simulink model "SimulinkAnalysisofCheetahTail"  (R2022a)
settings: Solver=ode4  StartTime=0.0  StopTime=1.5  FixedStep=0.001  RelTol=1e-3
undefined symbols (not defined in the file): B_cg_H, B_con_H, B_con_L, bar_len, cd_table, Cf, cl_table, g, gear_ratio, int_point_bar, int_point_tail, ITail, M_add, M_cg_H, M_cg_L, M_cg_W, Mb, Mm, Mt, psi3, rho, T_cg_H, T_fur_gap, T_length, T_width_major, T_width_minor, th2_initial, torque_constant, uncertainty_Forces, uncertainty_Position, Vf, windspeed
(part 10 of 21)

== matlab function SimulinkAnalysisofCheetahTail/Model/MassMatrix ==
  data: B_cg_H parameter; B_con_H parameter; B_con_L parameter; ITail parameter; M_cg_H parameter; M_cg_L parameter; M_cg_W parameter; Mb parameter; Mm parameter; Mt parameter; T_cg_H parameter; MassMatrix output; q input
function MassMatrix = MassMatrix(B_cg_H,B_con_H,B_con_L,ITail,M_cg_H,M_cg_L,M_cg_W,Mb,Mm,Mt,T_cg_H,q)
%#codegen
[x,y,z,phi1,th1,psi1,phi2,th2] = deal(q(1),q(2),q(3),q(4),q(5),q(6),q(7),q(8));
% [dx,dy,dz,dphi1,dth1,dpsi1,dphi2,dth2] = deal(dq(1),dq(2),dq(3),dq(4),dq(5),dq(6),dq(7),dq(8));
%    This function was generated by the Symbolic Math Toolbox version 9.0.
%    26-Jan-2022 10:16:26

t2 = cos(phi1);
t3 = cos(phi2);
t4 = cos(psi1);
t5 = cos(th1);
t6 = cos(th2);
t7 = sin(phi1);
t8 = sin(phi2);
t9 = sin(psi1);
t10 = sin(th1);
t11 = sin(th2);
t12 = M_cg_L+x;
t13 = M_cg_W+y;
t14 = M_cg_H+z;
t15 = B_cg_H.^2;
t16 = t2.^2;
t17 = t4.^2;
t18 = t5.^2;
t19 = t7.^2;
t20 = t9.^2;
t21 = t10.^2;
t22 = B_con_L.*t5;
t23 = t2.*t4;
t24 = t5.*t6;
t25 = t2.*t8;
t26 = t2.*t9;
t27 = t4.*t7;
t28 = t6.*t10;
t29 = t7.*t9;
t30 = t10.*t11;
t32 = t5.*t12;
t33 = B_con_H.*t2.*t10;
t34 = B_con_H.*t5.*t7;
t35 = B_con_L.*t4.*t10;
t37 = B_con_L.*t9.*t10;
t40 = t5.*t8.*t11;
t42 = t5.*t9.*t11;
t44 = t7.*t8.*t10;
t48 = t2.*t3.*t5;
t52 = t3.*t5.*t7;
t53 = t3.*t6.*t7;
t55 = t2.*t5.*t11;
t56 = t3.*t5.*t11;
t58 = t4.*t5.*t11;
t61 = t3.*t7.*t10;
t62 = t5.*t7.*t8;
t68 = t2.*t5.*t13;
t70 = t4.*t10.*t12;
t72 = Mb.*t2.*t5.*t10;
t73 = Mm.*t2.*t5.*t10;
t74 = Mt.*t2.*t5.*t10;
t75 = t2.*t10.*t14;
t76 = t5.*t7.*t14;
t77 = t9.*t10.*t12;
t78 = Mb.*t5.*t7.*t10;
t79 = Mm.*t5.*t7.*t10;
t80 = Mt.*t5.*t7.*t10;
t81 = t7.*t10.*t13;
t340 = t10.*7.84867146e-3;
t344 = t7.*1.19846373e-3;
t346 = t2.*3.949132625e-3;
t349 = t2.*1.0208097e-4;
t350 = t7.*1.0208097e-4;
t355 = t2.*t5.*1.19846373e-3;
t360 = t5.*t7.*3.949132625e-3;
t365 = t2.*4.699e-8;
t366 = t7.*1.8563e-7;
t367 = t7.*3.7126e-7;
t368 = t10.*1.8563e-7;
t371 = t2.*2.3495e-8;
t372 = t10.*2.3495e-8;
t376 = t2.*t5.*3.7126e-7;
t377 = t5.*t7.*4.699e-8;
t31 = t4.*t22;
t36 = t9.*t22;
t38 = t2.*t30;
t39 = t3.*t30;
t41 = t8.*t28;
t43 = t9.*t28;
t45 = t10.*t29;
t46 = t11.*t29;
t47 = t8.*t30;
t49 = t2.*t24;
t50 = t4.*t24;
t51 = t5.*t25;
t54 = t10.*t23;
t57 = t3.*t28;
t59 = t4.*t28;
t60 = t9.*t24;
t63 = t10.*t26;
t64 = t10.*t27;
t65 = t11.*t27;
t66 = B_con_H.*t5.*t23;
t67 = t4.*t32;
t69 = B_con_H.*t5.*t26;
t71 = t9.*t32;
t82 = -t33;
t83 = -t34;
t85 = -t44;
t90 = t11.*t48;
t92 = t24.*t25;
t93 = t3.*t7.*t24;
t94 = t5.*t11.*t23;
t95 = t4.*t56;
t97 = t5.*t8.*t27;
t99 = t25.*t28;
t100 = t7.*t8.*t24;
t101 = t23.*t30;
t102 = t5.*t11.*t26;
t104 = t3.*t42;
t105 = t4.*t40;
t106 = t5.*t8.*t29;
t108 = t26.*t30;
t110 = t9.*t40;
t112 = -t58;
t114 = t5.*t14.*t23;
t115 = t5.*t13.*t27;
t116 = t5.*t14.*t26;
t117 = t5.*t13.*t29;
t118 = -t68;
t120 = -t75;
t121 = -t76;
t122 = -t78;
t123 = -t79;
t124 = -t80;
t125 = Mb.*t2.*t7.*t18;
t126 = Mm.*t2.*t7.*t18;
t127 = Mt.*t2.*t7.*t18;
t128 = t3.*t23.*t24;
t129 = t3.*t24.*t26;
t140 = t44.*(2.7e+1./1.0e+2);
t142 = t25+t53;
t143 = t28+t55;
t149 = t52.*(2.7e+1./1.0e+2);
t150 = t56.*(2.7e+1./1.0e+2);
t194 = t68+t76;
t351 = -t344;
t354 = -t350;
t361 = t5.*t349;
t362 = t5.*t350;
t380 = -t372;
t388 = -t377;
t604 = -t2.*t5.*(t344-t349);
t620 = t366+t371;
t621 = t2.*t5.*(t344-t349);
t84 = -t38;
t86 = -t45;
t87 = -t47;
t88 = t3.*t49;
t89 = t3.*t50;
t91 = t2.*t57;
t96 = t3.*t60;
t98 = t11.*t51;
t103 = t4.*t39;
t107 = -t49;
t109 = t9.*t39;
t111 = -t54;
t113 = -t60;
t119 = -t71;
t131 = -t95;
t133 = -t100;
t134 = -t101;
t135 = -t115;
t136 = -t117;
t137 = -t125;
t138 = -t126;
t139 = -t127;
t141 = t47.*(2.7e+1./1.0e+2);
t144 = t26+t64;
t145 = t27+t63;
t146 = -t128;
t147 = -t129;
t148 = t51.*(2.7e+1./1.0e+2);
t151 = t57.*(2.7e+1./1.0e+2);
t152 = -t140;
t161 = t90.*(2.7e+1./1.0e+2);
t163 = t92.*(2.7e+1./1.0e+2);
t164 = t93.*(2.7e+1./1.0e+2);
t165 = t95.*(2.7e+1./1.0e+2);
t167 = t143.^2;
t168 = t97.*(2.7e+1./1.0e+2);
t172 = t104.*(2.7e+1./1.0e+2);
t173 = t105.*(2.7e+1./1.0e+2);
t174 = t106.*(2.7e+1./1.0e+2);
t176 = t110.*(2.7e+1./1.0e+2);
t184 = t51+t93;
t188 = t57+t90;
t189 = t59+t94;
t191 = t43+t102;
t192 = t128.*(2.7e+1./1.0e+2);
t193 = t129.*(2.7e+1./1.0e+2);
t240 = Mm.*t10.*t194;
t260 = Mm.*t2.*t5.*t194;
t261 = Mm.*t5.*t7.*t194;
t268 = t40+t61+t99;
t279 = t32+t81+t120;
t302 = t5.*t142.*t143;
t579 = t349+t351;
t581 = t346+t354;
t635 = t10.*t620;
t763 = t355+t362+t368;
t771 = t360+t361+t380;
t130 = -t88;
t132 = -t96;
t153 = -t141;
t154 = B_con_H.*t144;
t155 = B_con_H.*t145;
t156 = t24+t84;
t157 = t30+t107;
t158 = t23+t86;
t159 = t29+t111;
t160 = t89.*(2.7e+1./1.0e+2);
t162 = t91.*(2.7e+1./1.0e+2);
t166 = t96.*(2.7e+1./1.0e+2);
t169 = t144.^2;
t170 = t145.^2;
t171 = t103.*(2.7e+1./1.0e+2);
t175 = t109.*(2.7e+1./1.0e+2);
t177 = t3.*t144;
t178 = t3.*t145;
t179 = t6.*t145;
t180 = t8.*t144;
t181 = t8.*t145;
t182 = t11.*t145;
t190 = t41+t98;
t197 = t13.*t144;
t198 = t13.*t145;
t199 = t14.*t144;
t200 = t14.*t145;
t201 = t3.*t167;
t204 = -t192;
t208 = -t193;
t215 = t48+t133;
t216 = B_cg_H.*t184;
t217 = T_cg_H.*t184;
t218 = T_cg_H.*t188;
t219 = Mb.*t4.*t5.*t144;
t220 = Mm.*t4.*t5.*t144;
t221 = Mt.*t4.*t5.*t144;
t222 = Mb.*t5.*t9.*t145;
t223 = Mm.*t5.*t9.*t145;
t224 = Mt.*t5.*t9.*t145;
t259 = B_cg_H.*Mb.*t10.*t188;
t262 = -t240;
t274 = B_cg_H.*Mb.*t2.*t5.*t188;
t277 = B_cg_H.*Mb.*t5.*t7.*t188;
t278 = -t260;
t284 = t56+t85+t91;
t285 = t52+t87+t92;
t286 = t46+t50+t134;
t287 = t65+t108+t113;
t303 = Mm.*t10.*t279;
t312 = Mm.*t2.*t5.*t279;
t313 = Mm.*t5.*t7.*t279;
t314 = t70+t114+t135;
t315 = t77+t116+t136;
t317 = t302./2.0;
t320 = t97+t103+t146;
t321 = t106+t109+t147;
t374 = Mm.*t194.*t279;
t462 = t302.*3.36554e-3;
t475 = t302.*3.372786875e-3;
t476 = t302.*9.53094055e-4;
t601 = t5.*t7.*t581;
t775 = t7.*t763;
t781 = t2.*t771;
t183 = -t166;
t185 = B_con_H.*t158;
t186 = B_con_H.*t159;
t187 = -t155;
t195 = t158.^2;
t196 = t159.^2;
t202 = t6.*t177;
t203 = t6.*t178;
t205 = t11.*t178;
t206 = t6.*t180;
t207 = t8.*t179;
t209 = t3.*t158;
t210 = t3.*t159;
t211 = t6.*t159;
t212 = t8.*t158;
t213 = t8.*t159;
t214 = t11.*t159;
t225 = t13.*t158;
t226 = t13.*t159;
t227 = -t198;
t228 = t14.*t158;
t229 = t14.*t159;
t230 = -t199;
t231 = -t200;
t239 = t201./2.0;
t241 = -t216;
t242 = Mb.*t4.*t5.*t159;
t243 = Mm.*t4.*t5.*t159;
t244 = Mt.*t4.*t5.*t159;
t245 = Mb.*t5.*t9.*t158;
t246 = -t222;
t247 = Mm.*t5.*t9.*t158;
t248 = -t223;
t249 = Mt.*t5.*t9.*t158;
t250 = -t224;
t256 = t177.*(2.7e+1./1.0e+2);
t257 = t180.*(2.7e+1./1.0e+2);
t258 = t181.*(2.7e+1./1.0e+2);
t267 = t42+t179;
t282 = t113+t182;
t283 = t39+t62+t130;
t292 = -t277;
t298 = B_cg_H.*t284;
t299 = T_cg_H.*t284;
t300 = T_cg_H.*t285;
t304 = Mb.*t144.*t159;
t305 = Mb.*t145.*t158;
t306 = Mm.*t144.*t159;
t307 = Mm.*t145.*t158;
t308 = Mt.*t144.*t159;
t309 = Mt.*t145.*t158;
t316 = B_cg_H.*Mb.*t10.*t285;
t323 = t5.*t7.*t11.*t285;
t324 = -t313;
t325 = B_cg_H.*Mb.*t2.*t5.*t285;
t326 = B_cg_H.*Mb.*t5.*t7.*t285;
t327 = B_cg_H.*t320;
t328 = T_cg_H.*t320;
t329 = B_cg_H.*t321;
t330 = T_cg_H.*t321;
t333 = Mm.*t4.*t5.*t314;
t335 = Mm.*t5.*t9.*t315;
t352 = t143.*t284;
t353 = t143.*t285;
t363 = t156.*t285;
t364 = t157.*t285;
t385 = Mm.*t145.*t315;
t391 = -t374;
t392 = Mm.*t144.*t314;
t397 = Mm.*t158.*t315;
t406 = Mb.*t15.*t188.*t285;
t409 = Mm.*t159.*t314;
t411 = t151+t161+t218;
t414 = t201.*3.36554e-3;
t433 = t201.*3.372786875e-3;
t435 = t201.*9.53094055e-4;
t445 = -t3.*t287.*(t60-t182);
t459 = t3.*t287.*(t60-t182).*(-1.0./2.0);
t533 = t83+t118+t121+t148+t164+t217;
t566 = Mt.*t10.*(-t34+t148+t164-t194+t217);
t582 = Mt.*t2.*t5.*(-t34+t148+t164-t194+t217);
t583 = Mt.*t5.*t7.*(-t34+t148+t164-t194+t217);
t612 = t3.*t287.*(t60-t182).*(-3.36554e-3);
t616 = -t601;
t632 = t3.*t287.*(t60-t182).*(-3.372786875e-3);
t634 = t3.*t287.*(t60-t182).*(-9.53094055e-4);
t789 = -t781;
t232 = t6.*t209;
t233 = t6.*t210;
t234 = -t202;
t235 = t11.*t210;
t236 = t6.*t212;
t237 = t8.*t211;
t238 = -t209;
t251 = -t225;
t252 = -t226;
t253 = -t228;
t263 = -t257;
t264 = -t245;
t265 = -t247;
t266 = -t249;
t269 = t202.*(2.7e+1./1.0e+2);
t270 = t203.*(2.7e+1./1.0e+2);
t271 = t205.*(2.7e+1./1.0e+2);
t272 = t207.*(2.7e+1./1.0e+2);
t273 = t209.*(2.7e+1./1.0e+2);
t275 = t212.*(2.7e+1./1.0e+2);
t276 = t213.*(2.7e+1./1.0e+2);
t293 = t50+t214;
t297 = t283.^2;
t301 = t112+t211;
t311 = t132+t205;
t319 = -T_cg_H.*(t96-t205);
t331 = -t326;
t332 = t323./2.0;
t336 = -B_cg_H.*Mb.*t5.*t9.*(t96-t205);
t338 = t206+t210;
t339 = -t333;
t341 = -t335;
t343 = t226+t230;
t345 = B_cg_H.*Mb.*t5.*t9.*(t96-t205);
t357 = -B_cg_H.*(t202-t213);
t359 = -T_cg_H.*(t202-t213);
t369 = t352./2.0;
t370 = t353./2.0;
t373 = t190.*t283;
t375 = t34+t194+t241;
t378 = t67+t197+t229;
t382 = t363./2.0;
t383 = t364./2.0;
t386 = -B_cg_H.*Mb.*t145.*(t96-t205);
t387 = t104+t203+t212;
t389 = t215.*t283;
t393 = t119+t200+t225;
t399 = -B_cg_H.*Mb.*t158.*(t96-t205);
t410 = -t392;
t423 = -t409;
t424 = t268.*t283;
t430 = Mt.*t10.*t411;
t434 = Mt.*t2.*t5.*t411;
t436 = Mt.*t5.*t7.*t411;
t444 = -t9.*t283.*(t60-t182);
t456 = t9.*t283.*(t60-t182).*(-1.0./2.0);
t474 = t323.*3.36554e-3;
t477 = t22+t82+t279+t298;
t496 = t323.*3.367829185e-3;
t501 = t149+t153+t163+t300;
t502 = t323.*8.56645e-6;
t505 = t352.*3.36554e-3;
t506 = t353.*3.36554e-3;
t515 = t363.*3.36554e-3;
t516 = t364.*3.36554e-3;
t529 = t352.*3.372786875e-3;
t530 = t353.*3.372786875e-3;
t531 = t352.*9.53094055e-4;
t532 = t353.*9.53094055e-4;
t546 = t363.*3.367829185e-3;
t547 = t364.*3.367829185e-3;
t557 = t35+t66+t314+t327;
t564 = t37+t69+t315+t329;
t573 = t363.*8.56645e-6;
t574 = t364.*8.56645e-6;
t593 = -t583;
t611 = t9.*t283.*(t60-t182).*(-3.36554e-3);
t630 = t9.*t283.*(t60-t182).*(-3.372786875e-3);
t633 = t9.*t283.*(t60-t182).*(-9.53094055e-4);
t678 = t22+t82+t150+t152+t162+t279+t299;
t760 = Mt.*t411.*(-t34+t148+t164-t194+t217);
t765 = t37+t69+t174+t175+t208+t315+t330;
t767 = t35+t66+t168+t171+t204+t314+t328;
t817 = t72+t73+t74+t242+t243+t244+t246+t248+t250;
t882 = t137+t138+t139+t304+t305+t306+t307+t308+t309;
t254 = -t232;
t255 = -t237;
t280 = -t269;
t281 = -t273;
t288 = t232.*(2.7e+1./1.0e+2);
t289 = t233.*(2.7e+1./1.0e+2);
t290 = t235.*(2.7e+1./1.0e+2);
t291 = t237.*(2.7e+1./1.0e+2);
t310 = t89+t235;
t322 = t297./2.0;
t337 = t178+t236;
t342 = t198+t253;
t348 = t213+t234;
t379 = -Mm.*t4.*t5.*(t199+t252);
t390 = -t373;
t394 = Mm.*t4.*t5.*(t199+t252);
t395 = t373./2.0;
t398 = B_cg_H.*t387;
t400 = T_cg_H.*t387;
t401 = t131+t180+t233;
t403 = Mb.*t10.*t375;
t404 = t110+t207+t238;
t405 = -t389;
t408 = t387.^2;
t412 = t389./2.0;
t418 = Mb.*t2.*t5.*t375;
t419 = Mb.*t5.*t7.*t375;
t425 = Mm.*t5.*t9.*t378;
t431 = Mm.*t4.*t5.*t393;
t438 = -Mm.*t144.*(t199+t252);
t439 = t424./2.0;
t442 = t4.*t283.*t293;
t443 = t3.*t286.*t293;
t446 = -t436;
t448 = -Mm.*t159.*(t199+t252);
t450 = Mm.*t144.*(t199+t252);
t458 = Mm.*t159.*(t199+t252);
t461 = Mm.*t145.*t378;
t463 = t297.*3.36554e-3;
t464 = Mm.*t158.*t378;
t466 = Mm.*t144.*t393;
t469 = Mm.*t159.*t393;
t472 = B_cg_H.*Mb.*t188.*t375;
t473 = t297.*3.372816795e-3;
t478 = t297.*9.52624335e-4;
t481 = -t474;
t488 = -t293.*(t202-t213);
t495 = Mb.*t10.*t477;
t498 = t293.*(t202-t213).*(-1.0./2.0);
t500 = -t496;
t503 = Mb.*t2.*t5.*t477;
t504 = Mb.*t5.*t7.*t477;
t507 = -Mm.*t314.*(t199+t252);
t509 = t183+t271+t319;
t511 = t293.*t387;
t513 = B_cg_H.*Mb.*t285.*t375;
t518 = -t516;
t519 = Mt.*t10.*t501;
t522 = t9.*t285.*t387;
t525 = t8.*t287.*t387;
t534 = t373.*3.36554e-3;
t537 = Mt.*t2.*t5.*t501;
t538 = Mt.*t5.*t7.*t501;
MassMatrix = ft_1({B_cg_H,ITail,Mb,Mm,Mt,T_cg_H,t10,t105,t11,t122,t123,t124,t144,t145,t148,t15,t154,t158,t159,t16,t160,t164,t165,t166,t169,t17,t170,t172,t173,t176,t177,t18,t181,t182,t185,t186,t187,t188,t189,t19,t191,t194,t195,t196,t199,t2,t20,t201,t202,t205,t21,t211,t213,t217,t219,t220,t221,t227,t228,t231,t239,t251,t252,t254,t255,t256,t258,t259,t261,t262,t263,t264,t265,t266,t267,t270,t271,t272,t274,t275,t276,t278,t279,t280,t281,t283,t285,t286,t288,t289,t290,t291,t292,t293,t297,t302,t303,t31,t310,t312,t314,t315,t316,t317,t322,t323,t324,t325,t331,t332,t337,t338,t339,t34,t340,t341,t342,t344,t345,t349,t352,t353,t357,t359,t36,t363,t364,t365,t367,t369,t370,t373,t375,t376,t378,t382,t383,t385,t386,t387,t388,t389,t390,t391,t393,t394,t395,t397,t398,t399,t4,t400,t401,t403,t404,t405,t406,t408,t410,t411,t412,t414,t418,t419,t423,t424,t425,t430,t431,t433,t434,t435,t439,t442,t443,t444,t445,t446,t450,t456,t458,t459,t461,t462,t463,t464,t466,t469,t472,t473,t474,t475,t476,t477,t478,t481,t488,t495,t496,t498,t5,t500,t501,t502,t503,t504,t505,t506,t507,t511,t513,t515,t518,t519,t522,t525,t529,t530,t531,t532,t534,t537,t538,t546,t547,t557,t564,t566,t573,t574,t58,t581,t582,t593,t60,t611,t612,t616,t621,t630,t632,t633,t634,t635,t678,t7,t71,t760,t763,t765,t767,t771,t775,t789,t8,t817,t882,t9,t96});
end
function MassMatrix = ft_1(ct)
B_cg_H = ct{1};
ITail = ct{2};
Mb = ct{3};
Mm = ct{4};
Mt = ct{5};
T_cg_H = ct{6};
t10 = ct{7};
t105 = ct{8};
t11 = ct{9};
t122 = ct{10};
t123 = ct{11};
t124 = ct{12};
t144 = ct{13};
t145 = ct{14};
t148 = ct{15};
t15 = ct{16};
t154 = ct{17};
t158 = ct{18};
t159 = ct{19};
t16 = ct{20};
t160 = ct{21};
t164 = ct{22};
t165 = ct{23};
t166 = ct{24};
t169 = ct{25};
t17 = ct{26};
t170 = ct{27};
t172 = ct{28};
t173 = ct{29};
t176 = ct{30};
t177 = ct{31};
t18 = ct{32};
t181 = ct{33};
t182 = ct{34};
t185 = ct{35};
t186 = ct{36};
t187 = ct{37};
t188 = ct{38};
t189 = ct{39};
t19 = ct{40};
t191 = ct{41};
t194 = ct{42};
t195 = ct{43};
t196 = ct{44};
t199 = ct{45};
t2 = ct{46};
t20 = ct{47};
t201 = ct{48};
t202 = ct{49};
t205 = ct{50};
t21 = ct{51};
t211 = ct{52};
t213 = ct{53};
t217 = ct{54};
t219 = ct{55};
t220 = ct{56};
t221 = ct{57};
t227 = ct{58};
t228 = ct{59};
t231 = ct{60};
t239 = ct{61};
t251 = ct{62};
t252 = ct{63};
t254 = ct{64};
t255 = ct{65};
t256 = ct{66};
t258 = ct{67};
t259 = ct{68};
t261 = ct{69};
t262 = ct{70};
t263 = ct{71};
t264 = ct{72};
t265 = ct{73};
t266 = ct{74};
t267 = ct{75};
t270 = ct{76};
t271 = ct{77};
t272 = ct{78};
t274 = ct{79};
t275 = ct{80};
t276 = ct{81};
t278 = ct{82};
t279 = ct{83};
t280 = ct{84};
t281 = ct{85};
t283 = ct{86};
t285 = ct{87};
t286 = ct{88};
t288 = ct{89};
t289 = ct{90};
t290 = ct{91};
t291 = ct{92};
t292 = ct{93};
t293 = ct{94};
t297 = ct{95};
t302 = ct{96};
t303 = ct{97};
t31 = ct{98};
t310 = ct{99};
t312 = ct{100};
t314 = ct{101};
t315 = ct{102};
t316 = ct{103};
t317 = ct{104};
t322 = ct{105};
t323 = ct{106};
t324 = ct{107};
t325 = ct{108};
t331 = ct{109};
t332 = ct{110};
t337 = ct{111};
t338 = ct{112};
t339 = ct{113};
t34 = ct{114};
t340 = ct{115};
t341 = ct{116};
t342 = ct{117};
t344 = ct{118};
t345 = ct{119};
t349 = ct{120};
t352 = ct{121};
t353 = ct{122};
t357 = ct{123};
t359 = ct{124};
t36 = ct{125};
t363 = ct{126};
t364 = ct{127};
t365 = ct{128};
t367 = ct{129};
t369 = ct{130};
t370 = ct{131};
t373 = ct{132};
t375 = ct{133};
t376 = ct{134};
t378 = ct{135};
t382 = ct{136};
t383 = ct{137};
t385 = ct{138};
t386 = ct{139};
t387 = ct{140};
t388 = ct{141};
t389 = ct{142};
t390 = ct{143};
t391 = ct{144};
t393 = ct{145};
t394 = ct{146};
t395 = ct{147};
t397 = ct{148};
t398 = ct{149};
t399 = ct{150};
t4 = ct{151};
t400 = ct{152};
t401 = ct{153};
t403 = ct{154};
t404 = ct{155};
t405 = ct{156};
t406 = ct{157};
t408 = ct{158};
t410 = ct{159};
t411 = ct{160};
t412 = ct{161};
t414 = ct{162};
t418 = ct{163};
t419 = ct{164};
t423 = ct{165};
t424 = ct{166};
t425 = ct{167};
t430 = ct{168};
t431 = ct{169};
t433 = ct{170};
t434 = ct{171};
t435 = ct{172};
t439 = ct{173};
t442 = ct{174};
t443 = ct{175};
t444 = ct{176};
t445 = ct{177};
t446 = ct{178};
t450 = ct{179};
t456 = ct{180};
t458 = ct{181};
t459 = ct{182};
t461 = ct{183};
t462 = ct{184};
t463 = ct{185};
t464 = ct{186};
t466 = ct{187};
t469 = ct{188};
t472 = ct{189};
t473 = ct{190};
t474 = ct{191};
t475 = ct{192};
t476 = ct{193};
t477 = ct{194};
t478 = ct{195};
t481 = ct{196};
t488 = ct{197};
t495 = ct{198};
t496 = ct{199};
t498 = ct{200};
t5 = ct{201};
t500 = ct{202};
t501 = ct{203};
t502 = ct{204};
t503 = ct{205};
t504 = ct{206};
t505 = ct{207};
t506 = ct{208};
t507 = ct{209};
t511 = ct{210};
t513 = ct{211};
t515 = ct{212};
t518 = ct{213};
t519 = ct{214};
t522 = ct{215};
t525 = ct{216};
t529 = ct{217};
t530 = ct{218};
t531 = ct{219};
t532 = ct{220};
t534 = ct{221};
t537 = ct{222};
t538 = ct{223};
t546 = ct{224};
t547 = ct{225};
t557 = ct{226};
t564 = ct{227};
t566 = ct{228};
t573 = ct{229};
t574 = ct{230};
t58 = ct{231};
t581 = ct{232};
t582 = ct{233};
t593 = ct{234};
t60 = ct{235};
t611 = ct{236};
t612 = ct{237};
t616 = ct{238};
t621 = ct{239};
t630 = ct{240};
t632 = ct{241};
t633 = ct{242};
t634 = ct{243};
t635 = ct{244};
t678 = ct{245};
t7 = ct{246};
t71 = ct{247};
t760 = ct{248};
t763 = ct{249};
t765 = ct{250};
t767 = ct{251};
t771 = ct{252};
t775 = ct{253};
t789 = ct{254};
t8 = ct{255};
t817 = ct{256};
t882 = ct{257};
t9 = ct{258};
t96 = ct{259};
t545 = Mm.*t315.*t378;
t548 = t389.*3.36554e-3;
t558 = -t547;
t559 = -Mt.*t5.*t9.*(t166-t271+T_cg_H.*(t96-t205));
t571 = t373.*9.52624335e-4;
t572 = t373.*3.372816795e-3;
t575 = Mm.*t314.*t393;
t577 = Mt.*t5.*t9.*(t166-t271+T_cg_H.*(t96-t205));
t584 = t389.*9.52624335e-4;
t585 = t389.*3.372816795e-3;
t591 = t424.*3.36554e-3;
t596 = Mb.*t5.*t9.*t564;
t599 = Mb.*t4.*t5.*t557;
t600 = B_cg_H.*Mb.*t188.*t477;
t614 = t424.*9.52624335e-4;
t615 = t424.*3.372816795e-3;
t617 = -Mt.*t145.*(t166-t271+T_cg_H.*(t96-t205));
t619 = -Mm.*t393.*(t199+t252);
t624 = -Mt.*t158.*(t166-t271+T_cg_H.*(t96-t205));
t625 = Mm.*t393.*(t199+t252);
t638 = B_cg_H.*Mb.*t285.*t477;
t639 = Mb.*t145.*t564;
t640 = Mb.*t144.*t557;
t642 = t154+t199+t252+t357;
t643 = Mb.*t158.*t564;
t645 = Mb.*t159.*t557;
t650 = t293.*(t202-t213).*(-3.36554e-3);
t661 = t293.*(t202-t213).*(-3.372786875e-3);
t664 = t293.*(t202-t213).*(-9.53094055e-4);
t709 = Mt.*t10.*t678;
t712 = Mb.*t375.*t477;
t722 = -B_cg_H.*Mb.*t564.*(t96-t205);
t728 = Mt.*t2.*t5.*t678;
t729 = Mt.*t5.*t7.*t678;
t754 = Mt.*t411.*t501;
t785 = Mt.*t4.*t5.*t767;
t788 = Mt.*t5.*t9.*t765;
t803 = Mt.*t145.*t765;
t804 = Mt.*t144.*t767;
t805 = Mt.*t158.*t765;
t806 = Mt.*t159.*t767;
t814 = Mt.*t501.*(-t34+t148+t164-t194+t217);
t828 = t122+t123+t124+t219+t220+t221+t264+t265+t266;
t829 = Mt.*t411.*t678;
t846 = Mt.*t501.*t678;
t849 = Mt.*t678.*(-t34+t148+t164-t194+t217);
t871 = -Mt.*t765.*(t166-t271+T_cg_H.*(t96-t205));
t294 = -t288;
t295 = -t289;
t296 = -t291;
t318 = T_cg_H.*t310;
t334 = B_cg_H.*Mb.*t4.*t5.*t310;
t347 = t181+t254;
t381 = Mm.*t5.*t9.*t342;
t384 = B_cg_H.*Mb.*t144.*t310;
t396 = B_cg_H.*Mb.*t159.*t310;
t402 = t105+t177+t255;
t407 = -t395;
t413 = B_cg_H.*t401;
t415 = T_cg_H.*t401;
t417 = T_cg_H.*t404;
t420 = -t403;
t421 = -t412;
t422 = t401.^2;
t428 = t408./2.0;
t429 = -t418;
t437 = Mm.*t145.*t342;
t441 = B_cg_H.*Mb.*t5.*t9.*t404;
t447 = Mm.*t158.*t342;
t453 = -t442;
t454 = t442./2.0;
t455 = t443./2.0;
t465 = -t461;
t468 = -t464;
t471 = B_cg_H.*Mb.*t145.*t404;
t480 = t191.*t404;
t482 = t11.*t158.*t404;
t485 = B_cg_H.*Mb.*t158.*t404;
t487 = -t472;
t508 = Mm.*t315.*t342;
t510 = -t504;
t512 = t267.*t404;
t520 = -t401.*(t60-t182);
t524 = t293.*t404;
t526 = -t404.*(t60-t182);
t528 = -t513;
t535 = t511./2.0;
t539 = t4.*t285.*t401;
t540 = t8.*t286.*t401;
t542 = t401.*(t60-t182);
t551 = t522./2.0;
t554 = t525./2.0;
t555 = t404.*(t60-t182).*(-1.0./2.0);
t556 = -t538;
t560 = -t548;
t565 = -t545;
t576 = t408.*3.36554e-3;
t580 = -t571;
t586 = -t575;
t589 = -Mb.*t15.*t404.*(t96-t205);
t590 = -t584;
t592 = -t585;
t594 = t337.*t387;
t595 = t408.*9.52624335e-4;
t598 = t408.*3.372816795e-3;
t602 = t338.*t401;
t603 = Mm.*t342.*t378;
t606 = -t596;
t607 = t442.*3.36554e-3;
t609 = t443.*3.36554e-3;
t613 = -t599;
t627 = t442.*3.372786875e-3;
t628 = t443.*3.372786875e-3;
t629 = t442.*9.53094055e-4;
t631 = t443.*9.53094055e-4;
t646 = -t640;
t648 = t401.*t404;
t655 = -t645;
t659 = Mb.*t4.*t5.*t642;
t675 = t511.*3.36554e-3;
t681 = t522.*3.36554e-3;
t684 = t525.*3.36554e-3;
t685 = t404.*(t60-t182).*(-3.36554e-3);
t690 = t511.*9.53094055e-4;
t695 = t511.*3.372786875e-3;
t697 = Mb.*t144.*t642;
t701 = t522.*9.52624335e-4;
t704 = t525.*9.52624335e-4;
t705 = t522.*3.372816795e-3;
t706 = t404.*(t60-t182).*(-3.372786875e-3);
t707 = t525.*3.372816795e-3;
t708 = t404.*(t60-t182).*(-9.53094055e-4);
t716 = B_cg_H.*Mb.*t310.*t557;
t724 = Mb.*t159.*t642;
t731 = -t712;
t743 = -t729;
t749 = t36+t71+t187+t231+t251+t398;
t768 = B_cg_H.*Mb.*t310.*t642;
t770 = t201+t443+t445;
t774 = B_cg_H.*Mb.*t404.*t564;
t791 = -t785;
t794 = -t788;
t807 = -t804;
t808 = t154+t199+t252+t276+t280+t359;
t810 = -t806;
t843 = Mb.*t557.*t642;
t847 = t36+t71+t172+t187+t231+t251+t270+t275+t400;
t356 = B_cg_H.*t347;
t358 = T_cg_H.*t347;
t416 = T_cg_H.*t402;
t426 = -t413;
t427 = -t415;
t432 = t422./2.0;
t440 = B_cg_H.*Mb.*t4.*t5.*t402;
t449 = -t437;
t452 = -t441;
t457 = -t447;
t460 = -t454;
t467 = t11.*t144.*t402;
t470 = B_cg_H.*Mb.*t144.*t402;
t479 = -t347.*(t60-t182);
t483 = B_cg_H.*Mb.*t159.*t402;
t486 = t189.*t402;
t490 = -t482;
t492 = t347.*(t60-t182).*(-1.0./2.0);
t493 = t480./2.0;
t494 = t482./2.0;
t514 = t160+t290+t318;
t517 = -t508;
t521 = t293.*t402;
t523 = -t402.*(t60-t182);
t527 = -t512;
t536 = t512./2.0;
t541 = -t402.*(t58-t211);
t549 = t542.*(-1.0./2.0);
t552 = t402.*(t60-t182).*(-1.0./2.0);
t553 = t524./2.0;
t561 = -t539;
t562 = t542./2.0;
t568 = t539./2.0;
t569 = t540./2.0;
t570 = t402.*(t58-t211).*(-1.0./2.0);
t587 = t422.*3.36554e-3;
t588 = Mb.*t15.*t310.*t402;
t605 = t422.*9.52624335e-4;
t608 = t422.*3.372816795e-3;
t610 = t594./2.0;
t618 = -t607;
t623 = t602./2.0;
t636 = -t627;
t637 = -t629;
t641 = t387.*t402;
t651 = t347.*(t60-t182).*(-3.36554e-3);
t652 = t480.*3.36554e-3;
t654 = t482.*3.36554e-3;
t657 = t648./2.0;
t663 = t347.*(t60-t182).*(-3.372786875e-3);
t665 = t347.*(t60-t182).*(-9.53094055e-4);
t667 = t480.*3.367829185e-3;
t668 = t482.*3.367829185e-3;
t670 = t480.*8.56645e-6;
t671 = t482.*8.56645e-6;
t676 = t512.*3.36554e-3;
t677 = -t675;
t679 = t542.*(-3.36554e-3);
t682 = t402.*(t60-t182).*(-3.36554e-3);
t683 = t524.*3.36554e-3;
t687 = t402.*(t60-t182).*3.36554e-3;
t689 = -t684;
t691 = t512.*3.367829185e-3;
t692 = t539.*3.36554e-3;
t693 = t540.*3.36554e-3;
t694 = t402.*(t58-t211).*(-3.36554e-3);
t699 = t402.*(t58-t211).*3.36554e-3;
t700 = -t695;
t702 = t542.*(-9.53094055e-4);
t710 = t402.*(t60-t182).*(-3.367829185e-3);
t711 = t524.*3.367829185e-3;
t713 = t512.*8.56645e-6;
t714 = t542.*(-3.372786875e-3);
t717 = t542.*9.53094055e-4;
t719 = -t707;
t720 = t402.*(t60-t182).*3.367829185e-3;
t727 = t540.*3.372816795e-3;
t730 = t402.*(t58-t211).*(-3.367829185e-3);
t732 = t402.*(t60-t182).*(-8.56645e-6);
t733 = t524.*8.56645e-6;
t734 = t539.*9.52624335e-4;
t735 = t540.*9.52624335e-4;
t736 = t539.*3.372816795e-3;
t737 = -t716;
t739 = t402.*(t58-t211).*3.367829185e-3;
t745 = t176+t272+t281+t417;
t746 = t402.*(t58-t211).*(-8.56645e-6);
t747 = t594.*3.36554e-3;
t748 = t602.*3.36554e-3;
t750 = t594.*9.52624335e-4;
t751 = t594.*3.372816795e-3;
t756 = t602.*9.52624335e-4;
t757 = t602.*3.372816795e-3;
t762 = Mb.*t4.*t5.*t749;
t766 = t297+t408+t422;
t772 = t648.*3.36554e-3;
t777 = B_cg_H.*Mb.*t402.*t557;
t786 = t648.*9.52624335e-4;
t787 = t648.*3.372816795e-3;
t793 = Mb.*t144.*t749;
t797 = Mb.*t159.*t749;
t799 = t239+t455+t459;
t809 = B_cg_H.*Mb.*t402.*t642;
t815 = Mt.*t4.*t5.*t808;
t818 = t511+t542;
t820 = t352+t444+t453;
t822 = B_cg_H.*Mb.*t310.*t749;
t830 = Mt.*t144.*t808;
t833 = Mt.*t159.*t808;
t839 = B_cg_H.*Mb.*t402.*t749;
t845 = -t843;
t851 = Mt.*t4.*t5.*t847;
t860 = Mt.*t144.*t847;
t861 = t390+t525+t540;
t864 = Mt.*t159.*t847;
t867 = Mb.*t557.*t749;
t881 = Mb.*t642.*t749;
t885 = t405+t594+t602;
t892 = t435+t631+t634;
t906 = Mt.*t767.*t808;
t914 = -ITail.*t770.*(-t369+t454+(t9.*t283.*(t60-t182))./2.0);
t919 = -ITail.*t770.*(-t317+(t347.*(t60-t182))./2.0+(t293.*(t202-t213))./2.0);
t927 = Mt.*t767.*t847;
t937 = ITail.*(-t302+t347.*(t60-t182)+t293.*(t202-t213)).*(-t369+t454+(t9.*t283.*(t60-t182))./2.0);
t941 = ITail.*(-t317+(t347.*(t60-t182))./2.0+(t293.*(t202-t213))./2.0).*(-t352+t442+t9.*t283.*(t60-t182));
t944 = Mt.*t808.*t847;
t992 = -t770.*(-t531+t629+t9.*t283.*(t60-t182).*9.53094055e-4);
t998 = -t770.*(-t476+t347.*(t60-t182).*9.53094055e-4+t293.*(t202-t213).*9.53094055e-4);
t1019 = (-t302+t347.*(t60-t182)+t293.*(t202-t213)).*(-t531+t629+t9.*t283.*(t60-t182).*9.53094055e-4);
t1021 = (-t352+t442+t9.*t283.*(t60-t182)).*(-t476+t347.*(t60-t182).*9.53094055e-4+t293.*(t202-t213).*9.53094055e-4);
t1102 = t303+t339+t341+t495+t606+t613+t709+t791+t794;
t1106 = t312+t385+t423+t503+t639+t655+t728+t803+t810;
t1107 = t324+t397+t410+t510+t643+t646+t743+t805+t807;
t451 = -t440;
t484 = -t470;
t489 = t467./2.0;
t491 = -t483;
t497 = t486./2.0;
t499 = -t494;
t543 = -t521;
t544 = -t536;
t550 = t521./2.0;
t567 = Mt.*t4.*t5.*t514;
t578 = -t568;
t597 = -t588;
t622 = Mt.*t144.*t514;
t626 = Mt.*t159.*t514;
t644 = t467.*3.36554e-3;
t649 = t185+t227+t228+t356;
t653 = t641./2.0;
t656 = t486.*3.36554e-3;
t658 = t467.*3.367829185e-3;
t662 = t467.*8.56645e-6;
t666 = t486.*3.367829185e-3;
t672 = t486.*8.56645e-6;
t674 = -t671;
t680 = t521.*3.36554e-3;
t688 = -t683;
t696 = -t692;
t698 = -t693;
t703 = t521.*9.53094055e-4;
t715 = t521.*3.372786875e-3;
t721 = -t711;
t725 = -t713;
t738 = -t727;
t741 = -t734;
t742 = -t736;
t744 = t173+t256+t296+t416;
t752 = t31+t186+t378+t426;
t753 = Mt.*t5.*t9.*t745;
t764 = t641.*3.36554e-3;
t769 = -t762;
t778 = Mt.*t145.*t745;
t779 = t641.*9.52624335e-4;
t780 = t641.*3.372816795e-3;
t784 = Mt.*t158.*t745;
t798 = -t793;
t801 = -t797;
t802 = t322+t428+t432;
t811 = t185+t227+t228+t258+t294+t358;
t812 = -t809;
t816 = t523+t524;
t825 = -t822;
t826 = t535+t562;
t827 = t552+t553;
t831 = t369+t456+t460;
t834 = t302+t479+t488;
t836 = t323+t467+t490;
t838 = t317+t492+t498;
t842 = t363+t480+t486;
t850 = t31+t165+t186+t263+t295+t378+t427;
t852 = -Mt.*t745.*(t166-t271+T_cg_H.*(t96-t205));
t855 = -t851;
t858 = t641+t648;
t859 = t364+t527+t541;
t865 = -t860;
t872 = -t864;
t874 = Mt.*t514.*t767;
t878 = t424+t522+t561;
t879 = t407+t554+t569;
t884 = -t881;
t886 = Mt.*t514.*t808;
t889 = t690+t717;
t890 = t732+t733;
t891 = t421+t610+t623;
t893 = t478+t595+t605;
t894 = Mt.*t745.*t765;
t896 = Mt.*t514.*t847;
t897 = t531+t633+t637;
t905 = t476+t664+t665;
t908 = -t906;
t913 = ITail.*t799.*t818;
t916 = -ITail.*t799.*(-t352+t442+t9.*t283.*(t60-t182));
t920 = -ITail.*t799.*(-t302+t347.*(t60-t182)+t293.*(t202-t213));
t923 = t580+t704+t735;
t931 = -ITail.*t818.*(-t369+t454+(t9.*t283.*(t60-t182))./2.0);
t933 = ITail.*t818.*(-t369+t454+(t9.*t283.*(t60-t182))./2.0);
t936 = -ITail.*t818.*(-t317+(t347.*(t60-t182))./2.0+(t293.*(t202-t213))./2.0);
t939 = ITail.*t818.*(-t317+(t347.*(t60-t182))./2.0+(t293.*(t202-t213))./2.0);
t940 = t590+t750+t756;
t945 = -t944;
t948 = -ITail.*t799.*(-t353+t521+t404.*(t60-t182));
t976 = ITail.*(-t353+t521+t404.*(t60-t182)).*(-t369+t454+(t9.*t283.*(t60-t182))./2.0);
t980 = ITail.*(-t353+t521+t404.*(t60-t182)).*(-t317+(t347.*(t60-t182))./2.0+(t293.*(t202-t213))./2.0);
t991 = t818.*t892;
t994 = -t892.*(-t352+t442+t9.*t283.*(t60-t182));
t999 = -t892.*(-t302+t347.*(t60-t182)+t293.*(t202-t213));
t1007 = -t818.*(-t531+t629+t9.*t283.*(t60-t182).*9.53094055e-4);
t1008 = t818.*(-t531+t629+t9.*t283.*(t60-t182).*9.53094055e-4);
t1017 = -t818.*(-t476+t347.*(t60-t182).*9.53094055e-4+t293.*(t202-t213).*9.53094055e-4);
t1020 = t818.*(-t476+t347.*(t60-t182).*9.53094055e-4+t293.*(t202-t213).*9.53094055e-4);
t1028 = -t892.*(-t353+t521+t404.*(t60-t182));
t1043 = (-t353+t521+t404.*(t60-t182)).*(-t531+t629+t9.*t283.*(t60-t182).*9.53094055e-4);
t1052 = (-t353+t521+t404.*(t60-t182)).*(-t476+t347.*(t60-t182).*9.53094055e-4+t293.*(t202-t213).*9.53094055e-4);
t563 = -t550;
t647 = -t644;
t660 = -t658;
t669 = Mb.*t5.*t9.*t649;
t686 = -t680;
t718 = -t703;
t723 = Mb.*t145.*t649;
t726 = -t715;
t740 = Mb.*t158.*t649;
t755 = Mt.*t4.*t5.*t744;
t758 = -t753;
t761 = Mb.*t5.*t9.*t752;
t773 = -B_cg_H.*Mb.*t649.*(t96-t205);
t776 = Mt.*t144.*t744;
t782 = Mt.*t159.*t744;
t792 = Mb.*t145.*t752;
t795 = Mb.*t158.*t752;
t813 = B_cg_H.*Mb.*t404.*t649;
t819 = Mt.*t5.*t9.*t811;
t821 = -B_cg_H.*Mb.*t752.*(t96-t205);
t824 = B_cg_H.*Mb.*t752.*(t96-t205);
t832 = Mt.*t145.*t811;
t835 = Mt.*t158.*t811;
t837 = B_cg_H.*Mb.*t404.*t752;
t841 = t332+t489+t499;
t844 = Mb.*t564.*t649;
t848 = t382+t493+t497;
t853 = Mt.*t514.*t744;
t854 = Mt.*t5.*t9.*t850;
t856 = t353+t526+t543;
t862 = t653+t657;
t863 = Mt.*t145.*t850;
t868 = Mb.*t564.*t752;
t869 = Mt.*t158.*t850;
t873 = t383+t544+t570;
t877 = -t874;
t880 = t439+t551+t578;
t883 = Mb.*t649.*t752;
t888 = -Mt.*t811.*(t166-t271+T_cg_H.*(t96-t205));
t895 = Mt.*t744.*t767;
t898 = -Mt.*t850.*(t166-t271+T_cg_H.*(t96-t205));
t899 = Mt.*t744.*t808;
t900 = -t896;
t901 = Mt.*t850.*(t166-t271+T_cg_H.*(t96-t205));
t903 = Mt.*t745.*t811;
t904 = t779+t786;
t907 = Mt.*t765.*t811;
t909 = t502+t662+t674;
t910 = ITail.*t770.*t826;
t911 = t573+t670+t672;
t915 = -t913;
t917 = Mt.*t744.*t847;
t921 = Mt.*t745.*t850;
t924 = t574+t725+t746;
t925 = -ITail.*t826.*(-t352+t442+t9.*t283.*(t60-t182));
t926 = t259+t334+t345+t430+t567+t577;
t928 = t614+t701+t741;
t929 = ITail.*t826.*(-t352+t442+t9.*t283.*(t60-t182));
t930 = Mt.*t765.*t850;
t934 = -ITail.*t826.*(-t302+t347.*(t60-t182)+t293.*(t202-t213));
t935 = ITail.*t826.*(-t302+t347.*(t60-t182)+t293.*(t202-t213));
t938 = ITail.*t827.*t836;
t946 = -ITail.*t770.*(-t370+t550+(t404.*(t60-t182))./2.0);
t947 = Mt.*t811.*t850;
t949 = ITail.*t802.*t858;
t950 = ITail.*t827.*t842;
t953 = ITail.*t766.*t879;
t957 = ITail.*t802.*t861;
t960 = ITail.*t802.*t878;
t961 = -ITail.*t826.*(-t353+t521+t404.*(t60-t182));
t963 = t770.*t889;
t964 = t274+t386+t396+t434+t617+t626;
t966 = ITail.*t826.*(-t353+t521+t404.*(t60-t182));
t969 = -ITail.*t818.*(-t370+t550+(t404.*(t60-t182))./2.0);
t970 = -ITail.*t827.*(-t364+t512+t402.*(t58-t211));
t972 = t292+t384+t399+t446+t622+t624;
t973 = ITail.*t818.*(-t370+t550+(t404.*(t60-t182))./2.0);
t974 = ITail.*t766.*t891;
t975 = ITail.*(-t370+t550+(t404.*(t60-t182))./2.0).*(-t352+t442+t9.*t283.*(t60-t182));
t977 = -ITail.*t816.*(-t383+t536+(t402.*(t58-t211))./2.0);
t978 = ITail.*t802.*t885;
t979 = ITail.*(-t370+t550+(t404.*(t60-t182))./2.0).*(-t302+t347.*(t60-t182)+t293.*(t202-t213));
t982 = -ITail.*t836.*(-t383+t536+(t402.*(t58-t211))./2.0);
t983 = -t889.*(-t352+t442+t9.*t283.*(t60-t182));
t984 = t889.*(-t352+t442+t9.*t283.*(t60-t182));
t985 = -ITail.*t842.*(-t383+t536+(t402.*(t58-t211))./2.0);
t987 = ITail.*t842.*(-t383+t536+(t402.*(t58-t211))./2.0);
t989 = -t889.*(-t302+t347.*(t60-t182)+t293.*(t202-t213));
t990 = t889.*(-t302+t347.*(t60-t182)+t293.*(t202-t213));
t993 = -t991;
t996 = t836.*t890;
t1001 = ITail.*t858.*t879;
t1002 = t842.*t890;
t1009 = ITail.*t878.*t879;
t1011 = -t889.*(-t353+t521+t404.*(t60-t182));
t1014 = t889.*(-t353+t521+t404.*(t60-t182));
t1016 = ITail.*t858.*t891;
t1018 = -t890.*(-t364+t512+t402.*(t58-t211));
t1022 = ITail.*t879.*t885;
t1023 = ITail.*t861.*t891;
t1026 = -t770.*(-t532+t703+t404.*(t60-t182).*9.53094055e-4);
t1029 = t858.*t893;
t1030 = t766.*t923;
t1031 = ITail.*t878.*t891;
t1034 = t861.*t893;
t1039 = t878.*t893;
t1040 = -t818.*(-t532+t703+t404.*(t60-t182).*9.53094055e-4);
t1041 = t818.*(-t532+t703+t404.*(t60-t182).*9.53094055e-4);
t1042 = (-t532+t703+t404.*(t60-t182).*9.53094055e-4).*(-t352+t442+t9.*t283.*(t60-t182));
t1044 = t766.*t940;
t1048 = t885.*t893;
t1050 = -t816.*(-t574+t713+t402.*(t58-t211).*8.56645e-6);
t1051 = (-t302+t347.*(t60-t182)+t293.*(t202-t213)).*(-t532+t703+t404.*(t60-t182).*9.53094055e-4);
t1058 = -t836.*(-t574+t713+t402.*(t58-t211).*8.56645e-6);
t1059 = -t842.*(-t574+t713+t402.*(t58-t211).*8.56645e-6);
t1062 = t842.*(-t574+t713+t402.*(t58-t211).*8.56645e-6);
t1064 = t858.*t923;
t1070 = t878.*t923;
t1074 = t858.*t940;
MassMatrix = ft_2({ITail,Mb,Mm,Mt,T_cg_H,t10,t1001,t1002,t1008,t1009,t1014,t1016,t1018,t1019,t1020,t1021,t1022,t1023,t1026,t1028,t1029,t1030,t1031,t1034,t1039,t1041,t1042,t1043,t1044,t1048,t1050,t1051,t1052,t1058,t1062,t1064,t1070,t1074,t1102,t1106,t1107,t148,t15,t16,t164,t166,t169,t17,t170,t18,t182,t188,t19,t194,t195,t196,t199,t2,t20,t202,t205,t21,t211,t213,t217,t252,t261,t262,t271,t278,t279,t283,t285,t293,t302,t310,t314,t315,t316,t317,t325,t331,t34,t340,t342,t344,t347,t349,t352,t353,t364,t365,t367,t369,t370,t375,t376,t378,t381,t383,t388,t391,t393,t394,t402,t404,t406,t411,t414,t419,t420,t425,t429,t431,t433,t442,t449,t450,t451,t452,t454,t457,t458,t462,t463,t465,t466,t468,t469,t471,t473,t474,t475,t476,t477,t481,t484,t485,t487,t491,t496,t5,t500,t501,t505,t506,t507,t512,t514,t515,t517,t518,t519,t521,t528,t529,t530,t531,t532,t534,t536,t537,t542,t546,t548,t550,t555,t556,t557,t558,t560,t563,t564,t565,t566,t572,t574,t576,t58,t581,t582,t585,t586,t587,t589,t591,t592,t593,t597,t598,t60,t600,t603,t608,t609,t611,t612,t615,t616,t618,t621,t625,t628,t629,t630,t632,t635,t636,t638,t642,t644,t647,t649,t650,t651,t652,t654,t656,t658,t659,t660,t661,t663,t666,t667,t668,t669,t675,t676,t677,t678,t679,t681,t682,t683,t685,t686,t687,t688,t689,t691,t695,t696,t697,t698,t699,t7,t700,t703,t705,t706,t708,t710,t711,t713,t714,t718,t719,t720,t721,t722,t723,t724,t726,t731,t737,t738,t739,t740,t742,t744,t745,t747,t748,t749,t751,t752,t754,t755,t757,t758,t760,t761,t763,t764,t765,t766,t767,t768,t769,t770,t771,t772,t773,t774,t775,t776,t777,t778,t780,t782,t784,t787,t789,t792,t795,t798,t799,t801,t802,t808,t811,t812,t813,t814,t815,t816,t817,t818,t819,t824,t825,t826,t827,t828,t829,t830,t832,t833,t835,t836,t837,t839,t841,t842,t844,t845,t846,t847,t848,t849,t850,t852,t853,t854,t855,t858,t861,t862,t863,t865,t867,t868,t869,t871,t872,t877,t878,t879,t880,t882,t883,t884,t885,t886,t888,t889,t890,t891,t892,t893,t894,t895,t899,t9,t900,t901,t903,t904,t907,t908,t909,t910,t911,t914,t915,t916,t917,t919,t920,t921,t923,t926,t927,t928,t929,t930,t933,t935,t937,t938,t939,t940,t941,t945,t946,t947,t948,t949,t950,t953,t957,t96,t960,t963,t964,t966,t970,t972,t973,t974,t975,t976,t977,t978,t979,t980,t982,t984,t987,t990,t992,t993,t994,t996,t998,t999});
end
function MassMatrix = ft_2(ct)
ITail = ct{1};
Mb = ct{2};
Mm = ct{3};
Mt = ct{4};
T_cg_H = ct{5};
t10 = ct{6};
t1001 = ct{7};
t1002 = ct{8};
t1008 = ct{9};
t1009 = ct{10};
t1014 = ct{11};
t1016 = ct{12};
t1018 = ct{13};
t1019 = ct{14};
t1020 = ct{15};
t1021 = ct{16};
t1022 = ct{17};
t1023 = ct{18};
t1026 = ct{19};
t1028 = ct{20};
t1029 = ct{21};
t1030 = ct{22};
t1031 = ct{23};
t1034 = ct{24};
t1039 = ct{25};
t1041 = ct{26};
t1042 = ct{27};
t1043 = ct{28};
t1044 = ct{29};
t1048 = ct{30};
t1050 = ct{31};
t1051 = ct{32};
t1052 = ct{33};
t1058 = ct{34};
t1062 = ct{35};
t1064 = ct{36};
t1070 = ct{37};
t1074 = ct{38};
t1102 = ct{39};
t1106 = ct{40};
t1107 = ct{41};
t148 = ct{42};
t15 = ct{43};
t16 = ct{44};
t164 = ct{45};
t166 = ct{46};
t169 = ct{47};
t17 = ct{48};
t170 = ct{49};
t18 = ct{50};
t182 = ct{51};
t188 = ct{52};
t19 = ct{53};
t194 = ct{54};
t195 = ct{55};
t196 = ct{56};
t199 = ct{57};
t2 = ct{58};
t20 = ct{59};
t202 = ct{60};
t205 = ct{61};
t21 = ct{62};
t211 = ct{63};
t213 = ct{64};
t217 = ct{65};
t252 = ct{66};
t261 = ct{67};
t262 = ct{68};
t271 = ct{69};
t278 = ct{70};
t279 = ct{71};
t283 = ct{72};
t285 = ct{73};
t293 = ct{74};
t302 = ct{75};
t310 = ct{76};
t314 = ct{77};
t315 = ct{78};
t316 = ct{79};
t317 = ct{80};
t325 = ct{81};
t331 = ct{82};
t34 = ct{83};
t340 = ct{84};
t342 = ct{85};
t344 = ct{86};
t347 = ct{87};
t349 = ct{88};
t352 = ct{89};
t353 = ct{90};
t364 = ct{91};
t365 = ct{92};
t367 = ct{93};
t369 = ct{94};
t370 = ct{95};
t375 = ct{96};
t376 = ct{97};
t378 = ct{98};
t381 = ct{99};
t383 = ct{100};
t388 = ct{101};
t391 = ct{102};
t393 = ct{103};
t394 = ct{104};
t402 = ct{105};
t404 = ct{106};
t406 = ct{107};
t411 = ct{108};
t414 = ct{109};
t419 = ct{110};
t420 = ct{111};
t425 = ct{112};
t429 = ct{113};
t431 = ct{114};
t433 = ct{115};
t442 = ct{116};
t449 = ct{117};
t450 = ct{118};
t451 = ct{119};
t452 = ct{120};
t454 = ct{121};
t457 = ct{122};
t458 = ct{123};
t462 = ct{124};
t463 = ct{125};
t465 = ct{126};
t466 = ct{127};
t468 = ct{128};
t469 = ct{129};
t471 = ct{130};
t473 = ct{131};
t474 = ct{132};
t475 = ct{133};
t476 = ct{134};
t477 = ct{135};
t481 = ct{136};
t484 = ct{137};
t485 = ct{138};
t487 = ct{139};
t491 = ct{140};
t496 = ct{141};
t5 = ct{142};
t500 = ct{143};
t501 = ct{144};
t505 = ct{145};
t506 = ct{146};
t507 = ct{147};
t512 = ct{148};
t514 = ct{149};
t515 = ct{150};
t517 = ct{151};
t518 = ct{152};
t519 = ct{153};
t521 = ct{154};
t528 = ct{155};
t529 = ct{156};
t530 = ct{157};
t531 = ct{158};
t532 = ct{159};
t534 = ct{160};
t536 = ct{161};
t537 = ct{162};
t542 = ct{163};
t546 = ct{164};
t548 = ct{165};
t550 = ct{166};
t555 = ct{167};
t556 = ct{168};
t557 = ct{169};
t558 = ct{170};
t560 = ct{171};
t563 = ct{172};
t564 = ct{173};
t565 = ct{174};
t566 = ct{175};
t572 = ct{176};
t574 = ct{177};
t576 = ct{178};
t58 = ct{179};
t581 = ct{180};
t582 = ct{181};
t585 = ct{182};
t586 = ct{183};
t587 = ct{184};
t589 = ct{185};
t591 = ct{186};
t592 = ct{187};
t593 = ct{188};
t597 = ct{189};
t598 = ct{190};
t60 = ct{191};
t600 = ct{192};
t603 = ct{193};
t608 = ct{194};
t609 = ct{195};
t611 = ct{196};
t612 = ct{197};
t615 = ct{198};
t616 = ct{199};
t618 = ct{200};
t621 = ct{201};
t625 = ct{202};
t628 = ct{203};
t629 = ct{204};
t630 = ct{205};
t632 = ct{206};
t635 = ct{207};
t636 = ct{208};
t638 = ct{209};
t642 = ct{210};
t644 = ct{211};
t647 = ct{212};
t649 = ct{213};
t650 = ct{214};
t651 = ct{215};
t652 = ct{216};
t654 = ct{217};
t656 = ct{218};
t658 = ct{219};
t659 = ct{220};
t660 = ct{221};
t661 = ct{222};
t663 = ct{223};
t666 = ct{224};
t667 = ct{225};
t668 = ct{226};
t669 = ct{227};
t675 = ct{228};
t676 = ct{229};
t677 = ct{230};
t678 = ct{231};
t679 = ct{232};
t681 = ct{233};
t682 = ct{234};
t683 = ct{235};
t685 = ct{236};
t686 = ct{237};
t687 = ct{238};
t688 = ct{239};
t689 = ct{240};
t691 = ct{241};
t695 = ct{242};
t696 = ct{243};
t697 = ct{244};
t698 = ct{245};
t699 = ct{246};
t7 = ct{247};
t700 = ct{248};
t703 = ct{249};
t705 = ct{250};
t706 = ct{251};
t708 = ct{252};
t710 = ct{253};
t711 = ct{254};
t713 = ct{255};
t714 = ct{256};
t718 = ct{257};
t719 = ct{258};
t720 = ct{259};
t721 = ct{260};
t722 = ct{261};
t723 = ct{262};
t724 = ct{263};
t726 = ct{264};
t731 = ct{265};
t737 = ct{266};
t738 = ct{267};
t739 = ct{268};
t740 = ct{269};
t742 = ct{270};
t744 = ct{271};
t745 = ct{272};
t747 = ct{273};
t748 = ct{274};
t749 = ct{275};
t751 = ct{276};
t752 = ct{277};
t754 = ct{278};
t755 = ct{279};
t757 = ct{280};
t758 = ct{281};
t760 = ct{282};
t761 = ct{283};
t763 = ct{284};
t764 = ct{285};
t765 = ct{286};
t766 = ct{287};
t767 = ct{288};
t768 = ct{289};
t769 = ct{290};
t770 = ct{291};
t771 = ct{292};
t772 = ct{293};
t773 = ct{294};
t774 = ct{295};
t775 = ct{296};
t776 = ct{297};
t777 = ct{298};
t778 = ct{299};
t780 = ct{300};
t782 = ct{301};
t784 = ct{302};
t787 = ct{303};
t789 = ct{304};
t792 = ct{305};
t795 = ct{306};
t798 = ct{307};
t799 = ct{308};
t801 = ct{309};
t802 = ct{310};
t808 = ct{311};
t811 = ct{312};
t812 = ct{313};
t813 = ct{314};
t814 = ct{315};
t815 = ct{316};
t816 = ct{317};
t817 = ct{318};
t818 = ct{319};
t819 = ct{320};
t824 = ct{321};
t825 = ct{322};
t826 = ct{323};
t827 = ct{324};
t828 = ct{325};
t829 = ct{326};
t830 = ct{327};
t832 = ct{328};
t833 = ct{329};
t835 = ct{330};
t836 = ct{331};
t837 = ct{332};
t839 = ct{333};
t841 = ct{334};
t842 = ct{335};
t844 = ct{336};
t845 = ct{337};
t846 = ct{338};
t847 = ct{339};
t848 = ct{340};
t849 = ct{341};
t850 = ct{342};
t852 = ct{343};
t853 = ct{344};
t854 = ct{345};
t855 = ct{346};
t858 = ct{347};
t861 = ct{348};
t862 = ct{349};
t863 = ct{350};
t865 = ct{351};
t867 = ct{352};
t868 = ct{353};
t869 = ct{354};
t871 = ct{355};
t872 = ct{356};
t877 = ct{357};
t878 = ct{358};
t879 = ct{359};
t880 = ct{360};
t882 = ct{361};
t883 = ct{362};
t884 = ct{363};
t885 = ct{364};
t886 = ct{365};
t888 = ct{366};
t889 = ct{367};
t890 = ct{368};
t891 = ct{369};
t892 = ct{370};
t893 = ct{371};
t894 = ct{372};
t895 = ct{373};
t899 = ct{374};
t9 = ct{375};
t900 = ct{376};
t901 = ct{377};
t903 = ct{378};
t904 = ct{379};
t907 = ct{380};
t908 = ct{381};
t909 = ct{382};
t910 = ct{383};
t911 = ct{384};
t914 = ct{385};
t915 = ct{386};
t916 = ct{387};
t917 = ct{388};
t919 = ct{389};
t920 = ct{390};
t921 = ct{391};
t923 = ct{392};
t926 = ct{393};
t927 = ct{394};
t928 = ct{395};
t929 = ct{396};
t930 = ct{397};
t933 = ct{398};
t935 = ct{399};
t937 = ct{400};
t938 = ct{401};
t939 = ct{402};
t940 = ct{403};
t941 = ct{404};
t945 = ct{405};
t946 = ct{406};
t947 = ct{407};
t948 = ct{408};
t949 = ct{409};
t950 = ct{410};
t953 = ct{411};
t957 = ct{412};
t96 = ct{413};
t960 = ct{414};
t963 = ct{415};
t964 = ct{416};
t966 = ct{417};
t970 = ct{418};
t972 = ct{419};
t973 = ct{420};
t974 = ct{421};
t975 = ct{422};
t976 = ct{423};
t977 = ct{424};
t978 = ct{425};
t979 = ct{426};
t980 = ct{427};
t982 = ct{428};
t984 = ct{429};
t987 = ct{430};
t990 = ct{431};
t992 = ct{432};
t993 = ct{433};
t994 = ct{434};
t996 = ct{435};
t998 = ct{436};
t999 = ct{437};
t1077 = t861.*t940;
t1078 = t885.*t923;
t1082 = t878.*t940;
t1093 = t677+t679+t720+t721+t764+t772;
t1094 = t687+t688+t700+t714+t764+t772;
t1095 = t677+t679+t687+t688+t780+t787;
t1112 = t433+t518+t534+t628+t632+t676+t689+t698+t699;
t1113 = t414+t534+t558+t609+t612+t689+t691+t698+t739;
t1114 = t414+t518+t572+t609+t612+t676+t699+t719+t738;
t1115 = -t766.*(t542.*3.36554e-3+t675+t682+t683-t780-t787);
t1116 = -t770.*(t542.*3.372786875e-3+t682+t683+t695-t764-t772);
t1117 = t515+t529+t591+t630+t636+t652+t656+t681+t696;
t1118 = t505+t546+t591+t611+t618+t666+t667+t681+t696;
t1119 = t505+t515+t611+t615+t618+t652+t656+t705+t742;
t1123 = (-t352+t442+t9.*t283.*(t60-t182)).*(t542.*3.372786875e-3+t682+t683+t695-t764-t772);
t1124 = (-t302+t347.*(t60-t182)+t293.*(t202-t213)).*(t542.*3.372786875e-3+t682+t683+t695-t764-t772);
t1125 = -t836.*(t542.*3.36554e-3+t675+t710+t711-t764-t772);
t1126 = t836.*(t542.*3.36554e-3+t675+t710+t711-t764-t772);
t1127 = -t842.*(t542.*3.36554e-3+t675+t710+t711-t764-t772);
t1128 = (-t353+t521+t404.*(t60-t182)).*(t542.*3.372786875e-3+t682+t683+t695-t764-t772);
t1129 = (-t364+t512+t402.*(t58-t211)).*(t542.*3.36554e-3+t675+t710+t711-t764-t772);
t1131 = -t861.*(t542.*3.36554e-3+t675+t682+t683-t780-t787);
t1132 = t861.*(t542.*3.36554e-3+t675+t682+t683-t780-t787);
t1133 = -t878.*(t542.*3.36554e-3+t675+t682+t683-t780-t787);
t1134 = -t885.*(t542.*3.36554e-3+t675+t682+t683-t780-t787);
t1138 = -t766.*(-t462+t474+t585+t644-t654-t751-t757+t347.*(t60-t182).*3.36554e-3+t293.*(t202-t213).*3.36554e-3);
t1141 = -t770.*(t474-t475+t548+t644-t654-t747-t748+t347.*(t60-t182).*3.372786875e-3+t293.*(t202-t213).*3.372786875e-3);
t1153 = -t818.*(t474-t475+t548+t644-t654-t747-t748+t347.*(t60-t182).*3.372786875e-3+t293.*(t202-t213).*3.372786875e-3);
t1154 = -t816.*(-t462+t496+t548+t658-t668-t747-t748+t347.*(t60-t182).*3.36554e-3+t293.*(t202-t213).*3.36554e-3);
t1157 = t818.*(t474-t475+t548+t644-t654-t747-t748+t347.*(t60-t182).*3.372786875e-3+t293.*(t202-t213).*3.372786875e-3);
t1158 = (-t352+t442+t9.*t283.*(t60-t182)).*(t474-t475+t548+t644-t654-t747-t748+t347.*(t60-t182).*3.372786875e-3+t293.*(t202-t213).*3.372786875e-3);
t1159 = t816.*(-t462+t496+t548+t658-t668-t747-t748+t347.*(t60-t182).*3.36554e-3+t293.*(t202-t213).*3.36554e-3);
t1163 = -t842.*(-t462+t496+t548+t658-t668-t747-t748+t347.*(t60-t182).*3.36554e-3+t293.*(t202-t213).*3.36554e-3);
t1171 = -t858.*(-t462+t474+t585+t644-t654-t751-t757+t347.*(t60-t182).*3.36554e-3+t293.*(t202-t213).*3.36554e-3);
t1172 = (-t353+t521+t404.*(t60-t182)).*(t474-t475+t548+t644-t654-t747-t748+t347.*(t60-t182).*3.372786875e-3+t293.*(t202-t213).*3.372786875e-3);
t1173 = (-t364+t512+t402.*(t58-t211)).*(-t462+t496+t548+t658-t668-t747-t748+t347.*(t60-t182).*3.36554e-3+t293.*(t202-t213).*3.36554e-3);
t1176 = -t861.*(-t462+t474+t585+t644-t654-t751-t757+t347.*(t60-t182).*3.36554e-3+t293.*(t202-t213).*3.36554e-3);
t1177 = t861.*(-t462+t474+t585+t644-t654-t751-t757+t347.*(t60-t182).*3.36554e-3+t293.*(t202-t213).*3.36554e-3);
t1179 = -t878.*(-t462+t474+t585+t644-t654-t751-t757+t347.*(t60-t182).*3.36554e-3+t293.*(t202-t213).*3.36554e-3);
t673 = -t669;
t759 = -t755;
t783 = -t776;
t790 = -t782;
t796 = -t792;
t800 = -t795;
t823 = -t819;
t840 = -t837;
t857 = -t853;
t866 = t370+t555+t563;
t870 = -t863;
t875 = -t868;
t876 = -t869;
t887 = -t883;
t902 = -t899;
t912 = -t910;
t918 = t532+t708+t718;
t922 = -t921;
t932 = -t930;
t942 = ITail.*t816.*t841;
t943 = ITail.*t766.*t862;
t951 = -t947;
t952 = -t950;
t954 = ITail.*t816.*t848;
t955 = -t953;
t958 = -t957;
t959 = ITail.*t766.*t880;
t962 = ITail.*t841.*t842;
t965 = ITail.*t836.*t848;
t968 = -t963;
t981 = -ITail.*t841.*(-t364+t512+t402.*(t58-t211));
t986 = -ITail.*t848.*(-t364+t512+t402.*(t58-t211));
t988 = ITail.*t848.*(-t364+t512+t402.*(t58-t211));
t995 = t766.*t904;
t997 = ITail.*t861.*t862;
t1003 = -t1001;
t1004 = -t1002;
t1005 = ITail.*t862.*t878;
t1006 = ITail.*t858.*t880;
t1010 = ITail.*t861.*t880;
t1012 = -t1009;
t1015 = ITail.*t862.*t885;
t1024 = -t1022;
t1025 = -t1023;
t1027 = t816.*t909;
t1032 = ITail.*t880.*t885;
t1033 = -t1030;
t1035 = -t1034;
t1036 = t816.*t911;
t1037 = t766.*t928;
t1045 = t842.*t909;
t1046 = t836.*t911;
t1053 = t861.*t904;
t1056 = t878.*t904;
t1057 = -t909.*(-t364+t512+t402.*(t58-t211));
t1060 = t885.*t904;
t1061 = -t911.*(-t364+t512+t402.*(t58-t211));
t1063 = t911.*(-t364+t512+t402.*(t58-t211));
t1065 = -t1064;
t1066 = t858.*t928;
t1069 = t861.*t928;
t1071 = t463+t506+t576+t587+t685+t686;
t1073 = -t1070;
t1075 = t473+t506+t598+t608+t685+t686;
t1076 = t463+t530+t576+t587+t706+t726;
t1079 = -t1077;
t1080 = -t1078;
t1081 = t885.*t928;
t1103 = t425+t431+t761+t769+t854+t855;
t1110 = t261+t419+t450+t457+t593+t697+t740+t830+t835;
t1111 = t278+t429+t449+t458+t582+t723+t724+t832+t833;
t1120 = t475+t481+t560+t647+t654+t661+t663+t747+t748;
t1121 = t462+t500+t560+t650+t651+t660+t668+t747+t748;
t1122 = t462+t481+t592+t647+t650+t651+t654+t751+t757;
t1130 = -t1129;
t1135 = t766.*t1114;
t1136 = t766.*t1119;
t1137 = t770.*t1117;
t1139 = t818.*t1112;
t1140 = t816.*t1113;
t1143 = -t1112.*(-t352+t442+t9.*t283.*(t60-t182));
t1145 = t818.*t1117;
t1146 = t816.*t1118;
t1149 = -t1112.*(-t302+t347.*(t60-t182)+t293.*(t202-t213));
t1150 = t836.*t1113;
t1152 = -t1117.*(-t302+t347.*(t60-t182)+t293.*(t202-t213));
t1155 = t836.*t1118;
t1156 = t842.*t1113;
t1161 = t858.*t1114;
t1162 = -t1112.*(-t353+t521+t404.*(t60-t182));
t1164 = t858.*t1119;
t1165 = -t1117.*(-t353+t521+t404.*(t60-t182));
t1166 = -t1118.*(-t364+t512+t402.*(t58-t211));
t1167 = t878.*t1114;
t1168 = t1118.*(-t364+t512+t402.*(t58-t211));
t1169 = t861.*t1119;
t1174 = t885.*t1114;
t1175 = -t1173;
t1178 = t885.*t1119;
t956 = -t954;
t967 = -t962;
t971 = -t965;
t1000 = -t997;
t1013 = -t1010;
t1038 = -t1036;
t1047 = -t1045;
t1049 = -t1046;
t1054 = t316+t451+t452+t519+t758+t759;
t1055 = -t1053;
t1067 = t325+t471+t491+t537+t778+t790;
t1068 = t331+t484+t485+t556+t783+t784;
t1072 = -t1069;
t1083 = t770.*t1076;
t1084 = t816.*t1071;
t1086 = t818.*t1076;
t1088 = -t1076.*(-t352+t442+t9.*t283.*(t60-t182));
t1089 = t836.*t1071;
t1091 = -t1076.*(-t302+t347.*(t60-t182)+t293.*(t202-t213));
t1092 = t842.*t1071;
t1096 = -t1071.*(-t364+t512+t402.*(t58-t211));
t1097 = t1071.*(-t364+t512+t402.*(t58-t211));
t1098 = t858.*t1075;
t1099 = t861.*t1075;
t1101 = t878.*t1075;
t1104 = t885.*t1075;
t1105 = t262+t381+t394+t420+t566+t659+t673+t815+t823;
t1108 = t465+t469+t796+t801+t870+t872;
t1109 = t466+t468+t798+t800+t865+t876;
t1142 = -t1139;
t1144 = -t1140;
t1147 = -t1145;
t1148 = -t1146;
t1151 = -t1150;
t1160 = -t1155;
t1170 = -t1169;
t1186 = t340+t376+t388+t603+t625+t884+t887+t935+t938+t939+t942+t945+t951+t990+t996+t1015+t1016+t1020+t1027+t1060+t1074+t1124+t1126+t1134+t1157+t1159+t1171;
t1085 = -t1084;
t1087 = -t1086;
t1090 = -t1089;
t1100 = -t1099;
t1182 = t638+t774+t777+t846+t894+t895+t959+t960+t975+t976+t1037+t1039+t1042+t1043+t1088+t1092+t1101+t1136+t1165;
t1184 = t824+t825+t900+t901+t912+t915+t968+t970+t977+t993+t1000+t1003+t1018+t1050+t1055+t1065+t1116+t1130+t1132+t1142+t1144+t1161;
t1185 = t600+t722+t737+t829+t871+t877+t914+t916+t987+t988+t992+t994+t1012+t1013+t1062+t1063+t1072+t1073+t1137+t1143+t1156+t1167+t1168+t1170;
t1187 = t487+t760+t768+t773+t886+t888+t919+t920+t981+t982+t998+t999+t1024+t1025+t1057+t1058+t1079+t1080+t1141+t1149+t1151+t1174+t1175+t1177;
t1188 = t565+t586+t616+t621+t635+t775+t789+t867+t875+t927+t929+t932+t933+t952+t956+t984+t1004+t1005+t1006+t1008+t1038+t1056+t1066+t1123+t1127+t1133+t1147+t1148+t1164;
t1189 = t365+t367+t391+t507+t517+t731+t844+t845+t849+t907+t908+t937+t941+t967+t971+t1019+t1021+t1031+t1032+t1047+t1049+t1081+t1082+t1152+t1158+t1160+t1163+t1178+t1179;
t1180 = t839+t840+t917+t922+t943+t949+t966+t973+t995+t1014+t1029+t1041+t1085+t1087+t1098+t1115+t1128;
t1181 = t406+t589+t597+t754+t852+t857+t946+t948+t955+t958+t1026+t1028+t1033+t1035+t1083+t1097+t1100+t1135+t1162;
t1183 = t528+t812+t813+t814+t902+t903+t974+t978+t979+t980+t1044+t1048+t1051+t1052+t1090+t1091+t1104+t1138+t1172;
et1 = (-t302+t347.*(t60-t182)+t293.*(t202-t213)).*(-t476+t347.*(t60-t182).*9.53094055e-4+t293.*(t202-t213).*9.53094055e-4).*2.0+t836.*t909.*2.0+t885.*t940.*2.0+Mm.*(t199+t252).^2+Mt.*(-t34+t148+t164-t194+t217).^2+Mb.*t375.^2+Mb.*t642.^2+Mb.*t649.^2+Mm.*t194.^2+Mm.*t342.^2+Mt.*t808.^2+Mt.*t811.^2;
et2 = (-t302+t347.*(t60-t182)+t293.*(t202-t213)).*(t474-t475+t548+t644-t654-t747-t748+t347.*(t60-t182).*3.372786875e-3+t293.*(t202-t213).*3.372786875e-3).*2.0;
et3 = t836.*(-t462+t496+t548+t658-t668-t747-t748+t347.*(t60-t182).*3.36554e-3+t293.*(t202-t213).*3.36554e-3).*2.0;
et4 = t885.*(-t462+t474+t585+t644-t654-t751-t757+t347.*(t60-t182).*3.36554e-3+t293.*(t202-t213).*3.36554e-3).*-2.0+ITail.*t836.*t841.*2.0+ITail.*t885.*t891.*2.0+ITail.*(-t302+t347.*(t60-t182)+t293.*(t202-t213)).*(-t317+(t347.*(t60-t182))./2.0+(t293.*(t202-t213))./2.0).*2.0;
et5 = 7.84867146e-3;
et6 = t2.*t581.*2.0+t842.*t911.*2.0+t878.*t928.*2.0+t842.*t1118.*2.0+t878.*t1119.*2.0-t1117.*(-t352+t442+t9.*t283.*(t60-t182)).*2.0+t7.*(t344-t349).*2.0+Mb.*t477.^2+Mb.*t557.^2+Mb.*t564.^2+Mm.*t279.^2+Mm.*t314.^2+Mm.*t315.^2+Mt.*t678.^2+Mt.*t765.^2+Mt.*t767.^2+(-t352+t442+t9.*t283.*(t60-t182)).*(-t531+t629+t9.*t283.*(t60-t182).*9.53094055e-4).*2.0+ITail.*t842.*t848.*2.0+ITail.*t878.*t880.*2.0;
et7 = ITail.*(-t352+t442+t9.*t283.*(t60-t182)).*(-t369+t454+(t9.*t283.*(t60-t182))./2.0).*2.0;
et8 = t816.*(t542.*3.36554e-3+t675+t710+t711-t764-t772).*2.0-t858.*(t542.*3.36554e-3+t675+t682+t683-t780-t787).*2.0+t818.*(t542.*3.372786875e-3+t682+t683+t695-t764-t772).*2.0;
et9 = t10.*(t10.*3.92433573e-3+t2.*t5.*1.8563e-7-t5.*t7.*2.3495e-8).*2.0+t816.*t890.*2.0+t818.*t889.*2.0+t858.*t904.*2.0+Mb.*t749.^2+Mb.*t752.^2+Mm.*t378.^2+Mm.*t393.^2+Mt.*t847.^2+Mt.*t850.^2+ITail.*t816.*t827.*2.0+ITail.*t818.*t826.*2.0+ITail.*t858.*t862.*2.0+t2.*t5.*t763.*2.0+t5.*t7.*t771.*2.0;
mt1 = [Mb.*t21+Mm.*t21+Mt.*t21+Mb.*t17.*t18+Mb.*t18.*t20+Mm.*t17.*t18+Mm.*t18.*t20+Mt.*t17.*t18+Mt.*t18.*t20,t828,t817,t1105,t1102,t1103,t1054,t926,t828,Mb.*t169+Mb.*t195+Mm.*t169+Mm.*t195+Mt.*t169+Mt.*t195+Mb.*t18.*t19+Mm.*t18.*t19+Mt.*t18.*t19,t882,t1110,t1107,t1109,t1068,t972,t817,t882,Mb.*t170+Mb.*t196+Mm.*t170+Mm.*t196+Mt.*t170+Mt.*t196+Mb.*t16.*t18+Mm.*t16.*t18+Mt.*t16.*t18,t1111,t1106,t1108,t1067,t964,t1105,t1110,t1111,et1+et2+et3+et4+et5,t1189,t1186,t1183,t1187,t1102,t1107,t1106,t1189,et6+et7,t1188,t1182,t1185,t1103,t1109,t1108,t1186,t1188,et8+et9,t1180,t1184,t1054,t1068,t1067,t1183,t1182,t1180];
mt2 = [t766.*t893.*2.0+t766.*t1075.*2.0+Mt.*t501.^2+Mt.*t744.^2+Mt.*t745.^2+(-t353+t521+t404.*(t60-t182)).*(-t532+t703+t404.*(t60-t182).*9.53094055e-4).*2.0-t1076.*(-t353+t521+t404.*(t60-t182)).*2.0+ITail.*t766.*t802.*2.0+ITail.*(-t353+t521+t404.*(t60-t182)).*(-t370+t550+(t404.*(t60-t182))./2.0).*2.0+Mb.*t15.*t285.^2+Mb.*t15.*t402.^2+Mb.*t15.*t404.^2,t1181,t926,t972,t964,t1187,t1185,t1184,t1181];
mt3 = [Mt.*(t166-t271+T_cg_H.*(t96-t205)).^2+t770.*t892.*2.0+t861.*t923.*2.0+t770.*t1112.*2.0-t861.*t1114.*2.0+Mt.*t411.^2+Mt.*t514.^2+(-t574+t713+t402.*(t58-t211).*8.56645e-6).*(-t364+t512+t402.*(t58-t211)).*2.0+t1113.*(-t364+t512+t402.*(t58-t211)).*2.0+Mb.*t15.*(t96-t205).^2+ITail.*t770.*t799.*2.0+ITail.*t861.*t879.*2.0+ITail.*(-t364+t512+t402.*(t58-t211)).*(-t383+t536+(t402.*(t58-t211))./2.0).*2.0+Mb.*t15.*t188.^2+Mb.*t15.*t310.^2];
MassMatrix = reshape([mt1,mt2,mt3],8,8);
end
